simulink model "carcomplexsimulink"  (R2025b)
settings: Solver=FixedStepAuto  StartTime=0.0  StopTime=inf  FixedStep=0.05  RelTol=1e-3
libraries: robotlib x12
settings Model: Creator=sprinkle  LastModifiedBy=sprinkle
settings OptimizationCC: EnhancedBackFolding=on  PassReuseOutputArgsAs=Individual arguments  ZeroExternalMemoryAtStartup=off  ZeroInternalMemoryAtStartup=off  MaxStackSize=64  OptimizeBlockOrder=speed  DifferentSizesBufferReuse=on  OptimizationCustomize=off  EfficientTunableParamExpr=on
settings DebuggingCC: ParameterTunabilityLossMsg=error
settings HardwareCC: ProdBitPerPointer=32.0  ProdBitPerSizeT=32.0  ProdBitPerPtrDiffT=32.0  ProdLargestAtomicFloat=None  ProdIntDivRoundTo=Undefined  ProdEndianess=Unspecified  ProdWordSize=32.0  ProdHWDeviceType=Generic->Unspecified (assume 32-bit Generic)
settings SFSimCC: MATLABDynamicMemAlloc=off
settings RTWCC: SystemTargetFile=ert.tlc  HardwareBoard=Robot Operating System (ROS)  TLCOptions="-aInlineSetEventsForThisBaseRateFcn=TLC_FALSE -aSuppressMultiTaskScheduler=TLC_FALSE  -aRateBasedStepFcn=0"  GenCodeOnly=on  TemplateMakefile=ert_default_tmf  Toolchain=Catkin  TargetLang=C++  GPUComputeCapability=3.5  Description=Embedded Coder
settings CodeAppCC: ForceParamTrailComments=on  IgnoreCustomStorageClasses=off  OperatorAnnotations=on  SimulinkDataObjDesc=on  SFDataObjDesc=on  InsertBlockDesc=on
settings ERTTargetCC: InlinedParameterPlacement=Hierarchical  DynamicArrayContainerType=coder::array  SupportContinuousTime=on

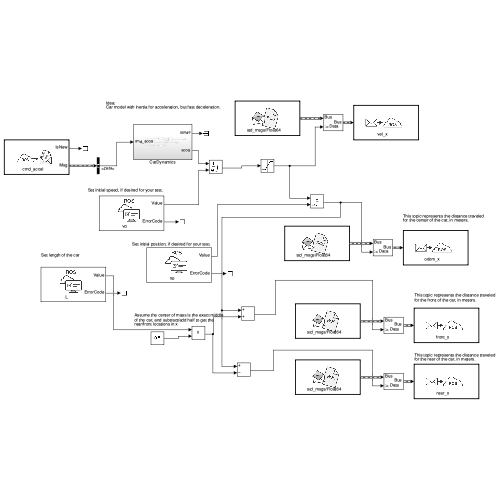
[thumbnail: Simulink's stored preview of the top-level diagram]
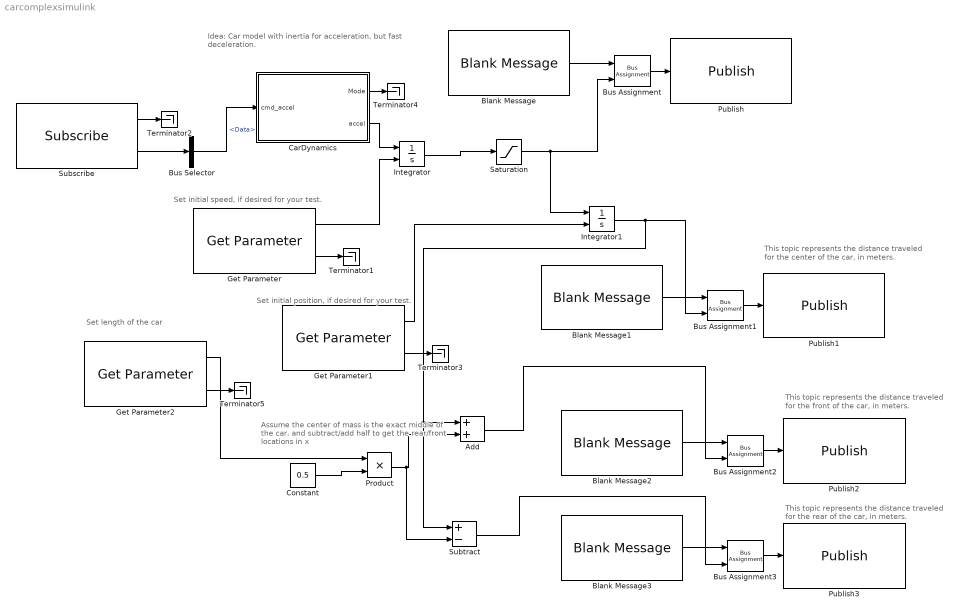
== system carcomplexsimulink ==
  note: Set length of the car
  note: This topic represents the distance traveled
      | for the center of the car, in meters.
  note: Set initial speed, if desired for your test.
  note: Idea:
      | Car model with inertia for acceleration, but fast deceleration.
  note: Set initial position, if desired for your test.
  note: This topic represents the distance traveled
      | for the front of the car, in meters.
  note: This topic represents the distance traveled
      | for the rear of the car, in meters.
  note: Assume the center of mass is the exact middle
      | of the car, and subtract/add half to get the
      | rear/front locations in x
  Add : Sum
  Blank Message{,1..3} (4 alike) : robotlib/Blank Message  messageClass=Message  entityType=std_msgs/Float64  messageType=std_msgs/Float64  SampleTime=inf  legacyBusStruct=off
      settings: LibrarySourceBlock=roslib/ROS/Blank Message
  Bus Assignment{,1..3} (4 alike) : BusAssignment  AssignedSignals=Data
  Bus Selector : BusSelector  OutputSignals=Data
  CarDynamics : Subsystem
  Constant : Constant  Value=0.5
  Get Parameter : robotlib/Get Parameter  ParameterSource=Specify your own  ParameterName=v0  ParameterType=double  ParameterMaxArrayLength=16  ParameterInitialValue=0.0  SampleTime=-1  ShowErrorCodeOutput=on  ModelName=carcomplexsimulink  BlockId=ParamGet_carcomplexsimulink_31
      settings: LibrarySourceBlock=roslib/ROS/Get Parameter
  Get Parameter1 : robotlib/Get Parameter  ParameterSource=Specify your own  ParameterName=x0  ParameterType=double  ParameterMaxArrayLength=16  ParameterInitialValue=0.0  SampleTime=-1  ShowErrorCodeOutput=on  ModelName=carcomplexsimulink  BlockId=ParamGet_carcomplexsimulink_37
      settings: LibrarySourceBlock=roslib/ROS/Get Parameter
  Get Parameter2 : robotlib/Get Parameter  ParameterSource=Specify your own  ParameterName=L  ParameterType=double  ParameterMaxArrayLength=16  ParameterInitialValue=4  SampleTime=-1  ShowErrorCodeOutput=on  ModelName=carcomplexsimulink  BlockId=ParamGet_carcomplexsimulink_50
      settings: LibrarySourceBlock=roslib/ROS/Get Parameter
  Integrator : Integrator  InitialConditionSource=external  LimitOutput=on  UpperSaturationLimit=40  LowerSaturationLimit=0
  Integrator1 : Integrator  InitialConditionSource=external
  Product : Product
  Publish : robotlib/Publish  topicSource=Specify your own  topic=vel_x  messageType=std_msgs/Float64  legacyBusStruct=off  messageQueueLength=1
      settings: LibrarySourceBlock=roslib/ROS/Publish
  Publish1 : robotlib/Publish  topicSource=Specify your own  topic=odom_x  messageType=std_msgs/Float64  legacyBusStruct=off  messageQueueLength=1
      settings: LibrarySourceBlock=roslib/ROS/Publish
  Publish2 : robotlib/Publish  topicSource=Specify your own  topic=front_x  messageType=std_msgs/Float64  legacyBusStruct=off  messageQueueLength=1
      settings: LibrarySourceBlock=roslib/ROS/Publish
  Publish3 : robotlib/Publish  topicSource=Specify your own  topic=rear_x  messageType=std_msgs/Float64  legacyBusStruct=off  messageQueueLength=1
      settings: LibrarySourceBlock=roslib/ROS/Publish
  Saturation : Saturate  UpperLimit=40  LowerLimit=0
  Subscribe : robotlib/Subscribe  topicSource=Specify your own  topic=cmd_accel  messageType=std_msgs/Float64  SampleTime=-1  legacyBusStruct=off  messageQueueLength=1
      settings: LibrarySourceBlock=roslib/ROS/Subscribe
  Subtract : Sum  Inputs=+-
  Terminator{1..5} (5 alike) : Terminator
  wires:
  Bus Selector/1 -> CarDynamics/1(cmd_accel)  "<Data>"
  CarDynamics/2(accel) -> Integrator/1
  Subscribe/1 -> Terminator2/1
  Integrator/1 -> Saturation/1
  Blank Message/1 -> Bus Assignment/1
  Bus Assignment/1 -> Publish/1
  Subscribe/2 -> Bus Selector/1
  Saturation/1 -> Integrator1/1, Bus Assignment/2
  Get Parameter/1 -> Integrator/2
  Get Parameter/2 -> Terminator1/1
  Blank Message1/1 -> Bus Assignment1/1
  Bus Assignment1/1 -> Publish1/1
  Integrator1/1 -> Subtract/1, Add/1, Bus Assignment1/2
  Get Parameter1/2 -> Terminator3/1
  Get Parameter1/1 -> Integrator1/2
  CarDynamics/1(Mode) -> Terminator4/1
  Get Parameter2/2 -> Terminator5/1
  Blank Message2/1 -> Bus Assignment2/1
  Add/1 -> Bus Assignment2/2
  Bus Assignment2/1 -> Publish2/1
  Bus Assignment3/1 -> Publish3/1
  Blank Message3/1 -> Bus Assignment3/1
  Subtract/1 -> Bus Assignment3/2
  Constant/1 -> Product/2
  Get Parameter2/1 -> Product/1
  Product/1 -> Subtract/2, Add/2

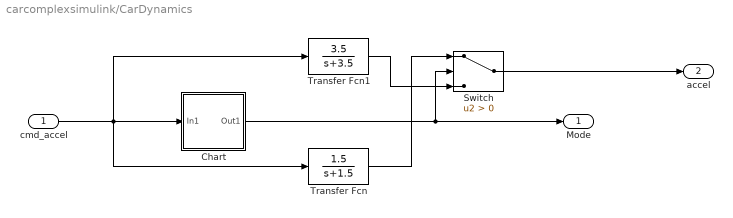
== system carcomplexsimulink/CarDynamics ==
  cmd_accel : Inport
  Chart : Stateflow chart  TreatAsAtomicUnit=on
  Switch : Switch  Criteria=u2 > Threshold  SaturateOnIntegerOverflow=off  InputSameDT=off
  Transfer Fcn : TransferFcn  Numerator=[1.5]  Denominator=[1 1.5]
  Transfer Fcn1 : TransferFcn  Numerator=[3.5]  Denominator=[1 3.5]
  Mode : Outport
  accel : Outport  Port=2
  wires:
  cmd_accel/1 -> Chart/1(In1), Transfer Fcn/1, Transfer Fcn1/1
  Transfer Fcn1/1 -> Switch/3
  Switch/1 -> accel/1
  Transfer Fcn/1 -> Switch/1
  Chart/1(Out1) -> Mode/1, Switch/2

== stateflow chart carcomplexsimulink/CarDynamics/Chart ==
  state Default
    entry: Out1=1;
  state Slowing
    entry: Out1=-1;
  (default) -> Default
  Slowing -> Default : [In1 > 0]
  Default -> Slowing : [In1 < 0.2]
  data: In1 input; Out1 output
